simulink model "ballInaHoop_trajStab"  (R2017a)
settings: Solver=ode45  StartTime=0.0  StopTime=15  MaxStep=1e-3  RelTol=1e-3  EnableMultiTasking=on
undefined symbols (not defined in the file): Dpsi0, Dth0, prms, psi0, th0
libraries: simulink x1
settings Model: Creator=gurtnmar  LastModifiedBy=marti
settings SolverCC: AlgebraicLoopSolver=LineSearch
settings DataIOCC: LimitDataPoints=on  SaveFormat=Array
settings OptimizationCC: LifeSpan=inf
settings DebuggingCC: SFUnexpectedBacktrackingDiag=warning  SFNoUnconditionalDefaultTransitionDiag=warning  SFExecutionAtInitializationDiag=none
settings HardwareCC: ProdBitPerPointer=32  ProdBitPerSizeT=32  ProdBitPerPtrDiffT=32  ProdLargestAtomicFloat=None  ProdIntDivRoundTo=Undefined  ProdEndianess=Unspecified  ProdWordSize=32  ProdHWDeviceType=32-bit Generic
settings ModelReferenceCC: PropagateSignalLabelsOutOfModel=off
settings GRTTargetCC: TargetLangStandard=C89/C90 (ANSI)  GeneratePreprocessorConditionals=Disable all
settings ConfigComp: CovMetricSettings=dw  CovHtmlReporting=on  CovSaveCumulativeToWorkspaceVar=on  CovSaveSingleToWorkspaceVar=on  CovExternalEMLEnable=off

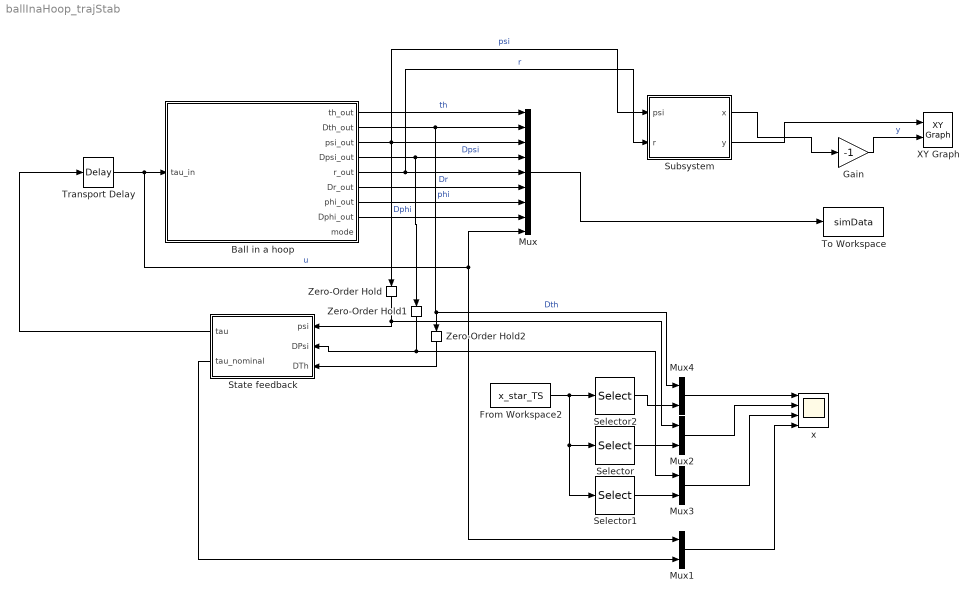
== system ballInaHoop_trajStab ==
  Ball in a hoop : Stateflow chart  TreatAsAtomicUnit=on
  From Workspace2 : FromWorkspace  VariableName=x_star_TS  SampleTime=prms.Ts  Interpolate=off  OutputAfterFinalValue=Setting to zero
  Gain : Gain  Gain=-1
  Mux : Mux  Inputs=9
  Mux{1..4} (4 alike) : Mux  Inputs=2
  Selector : Selector  InputPortWidth=3  IndexOptions=Index vector (dialog)  Indices=2  OutputSizes=1
  Selector1 : Selector  InputPortWidth=3  IndexOptions=Index vector (dialog)  Indices=3  OutputSizes=1
  Selector2 : Selector  InputPortWidth=3  IndexOptions=Index vector (dialog)  Indices=1  OutputSizes=1
  State feedback : Subsystem
  Subsystem : Subsystem
  To Workspace : ToWorkspace  VariableName=simData  SaveFormat=Timeseries  SampleTime=-1
  Transport Delay : TransportDelay  DelayTime=1/1000
  XY Graph : simulink/Sinks/XY Graph  xmin=-1.1*prms.Ro  xmax=1.1*prms.Ro  ymin=-1.1*prms.Ro  ymax=1.1*prms.Ro  st=-1
  Zero-Order Hold : ZeroOrderHold  SampleTime=prms.Ts
  Zero-Order Hold1 : ZeroOrderHold  SampleTime=prms.Ts
  Zero-Order Hold2 : ZeroOrderHold  SampleTime=prms.Ts
  x : Scope  NumInputPorts=4
  wires:
  Gain/1 -> XY Graph/2  "y"
  Mux/1 -> To Workspace/1
  Subsystem/2(y) -> XY Graph/1
  Subsystem/1(x) -> Gain/1
  Transport Delay/1 -> Ball in a hoop/1(tau_in), Mux/9, Mux1/1  "u"
  Ball in a hoop/1(th_out) -> Mux/1  "th"
  Ball in a hoop/2(Dth_out) -> Mux4/1, Zero-Order Hold2/1, Mux/2  "Dth"
  Ball in a hoop/3(psi_out) -> Zero-Order Hold/1, Subsystem/1(psi), Mux/3  "psi"
  Ball in a hoop/4(Dpsi_out) -> Zero-Order Hold1/1, Mux/4  "Dpsi"
  Ball in a hoop/5(r_out) -> Subsystem/2(r), Mux/5  "r"
  Ball in a hoop/6(Dr_out) -> Mux/6  "Dr"
  Ball in a hoop/7(phi_out) -> Mux/7  "phi"
  Ball in a hoop/8(Dphi_out) -> Mux/8  "Dphi"
  Zero-Order Hold1/1 -> Mux3/1, State feedback/2(DPsi)
  From Workspace2/1 -> Selector2/1, Selector1/1, Selector/1
  Selector/1 -> Mux2/2
  Selector1/1 -> Mux3/2
  Zero-Order Hold/1 -> Mux2/1, State feedback/1(psi)
  Mux4/1 -> x/1
  Mux2/1 -> x/2
  Mux3/1 -> x/3
  Selector2/1 -> Mux4/2
  Zero-Order Hold2/1 -> State feedback/3(DTh)
  Mux1/1 -> x/4
  State feedback/1(tau) -> Transport Delay/1
  State feedback/2(tau_nominal) -> Mux1/2

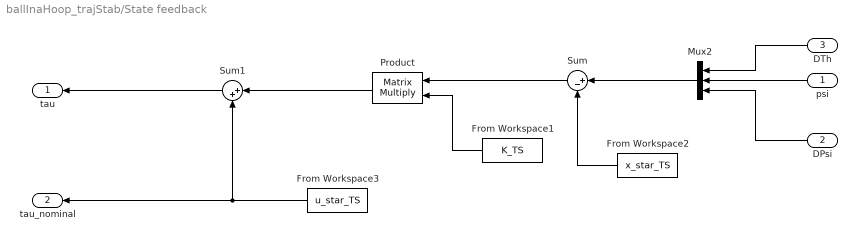
== system ballInaHoop_trajStab/State feedback ==
  psi : Inport
  DPsi : Inport  Port=2
  DTh : Inport  Port=3
  From Workspace1 : FromWorkspace  VariableName=K_TS  SampleTime=prms.Ts  Interpolate=off  OutputAfterFinalValue=Setting to zero
  From Workspace2 : FromWorkspace  VariableName=x_star_TS  SampleTime=prms.Ts  Interpolate=off  OutputAfterFinalValue=Setting to zero
  From Workspace3 : FromWorkspace  VariableName=u_star_TS  SampleTime=prms.Ts  Interpolate=off  OutputAfterFinalValue=Setting to zero
  Mux2 : Mux  Inputs=3
  Product : Product  Multiplication=Matrix(*)
  Sum : Sum  Inputs=|+-
  Sum1 : Sum  Inputs=|++
  tau : Outport
  tau_nominal : Outport  Port=2
  wires:
  From Workspace1/1 -> Product/2
  Mux2/1 -> Sum/1
  From Workspace2/1 -> Sum/2
  Sum1/1 -> tau/1
  psi/1 -> Mux2/2
  DPsi/1 -> Mux2/3
  Product/1 -> Sum1/1
  From Workspace3/1 -> Sum1/2, tau_nominal/1
  Sum/1 -> Product/1
  DTh/1 -> Mux2/1

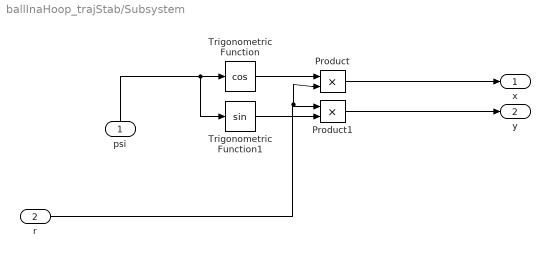
== system ballInaHoop_trajStab/Subsystem ==
  psi : Inport
  r : Inport  Port=2
  Product : Product
  Product1 : Product
  Trigonometric Function : Trigonometry  Operator=cos
  Trigonometric Function1 : Trigonometry
  x : Outport
  y : Outport  Port=2
  wires:
  Trigonometric Function/1 -> Product/1
  Product/1 -> x/1
  Product1/1 -> y/1
  Trigonometric Function1/1 -> Product1/2
  r/1 -> Product/2, Product1/1
  psi/1 -> Trigonometric Function1/1, Trigonometric Function/1

== stateflow chart ballInaHoop_trajStab/Ball in a hoop ==
  settings: updateMethod=CONTINUOUS
  state Free_fall
    du:
    th_dot = Dth;
    Dth_dot = prms.ath1*Dth + prms.bth*tau_in;
    phi_dot = Dphi;
    Dphi_dot = 0;
    r_dot = Dr;
    Dr_dot = r*Dpsi^2 + prms.g*cos(psi);
    psi_dot = Dpsi;
    Dpsi_dot = -(prms.g*sin(psi) + 2*Dpsi*Dr)/r;
    th_out = th;
    Dth_out = Dth;
    psi_out = psi;
    Dpsi_out = Dpsi;
    r_out = r;
    Dr_out = Dr;
    phi_out=phi;
    Dphi_out=Dphi;
    mode=2;
  state Ball_in_a_hoop
    du:
    th_dot = Dth;
    Dth_dot = prms.ath1*Dth + prms.ath2*sin(psi) + prms.ath3*Dpsi + prms.bth*tau_in;
    psi_dot = Dpsi;
    Dpsi_dot = prms.apsi1*Dth + prms.apsi2*sin(psi) + prms.apsi3*Dpsi + prms.bpsi*tau_in;
    th_out = th;
    Dth_out = Dth;
    psi_out = psi;
    Dpsi_out=Dpsi;
    phi_out=(th-psi)*prms.Ro/prms.Rb;
    Dphi_out = (Dth-Dpsi)*prms.Ro/prms.Rb;
    r_out = r;
    Dr_out = 0;
    mode=1;
  state Ball_on_the_inner_hoop
    du:
    th_dot = Dth;
    Dth_dot = prms.ath1*Dth + prms.bth*tau_in;
    psi_dot = Dpsi;
    Dpsi_dot = 1 / prms.in.a_bar * (-prms.in.b_bar*Dpsi ...
    - prms.in.c_bar*sin(psi) - prms.in.d_bar*Dth + prms.in.e_bar*tau_in);
    th_out = th;
    Dth_out = Dth;
    psi_out = psi;
    Dpsi_out=Dpsi;
    r_out = r;
    Dr_out = 0;
    phi_out= -(th-psi)*(prms.Ri/prms.Rb);
    Dphi_out = -(Dth-Dpsi)*(prms.Ri/prms.Rb);
    mode=3;
  (default) -> Ball_in_a_hoop : {
      | th=th0;
      | Dth=Dth0;
      | psi=psi0;
      | Dpsi=Dpsi0;
      | r = prms.Ro-prms.Rb;
      | }
  Ball_in_a_hoop -> Free_fall : [(-prms.g*cos(psi)-(prms.Ro-prms.Rb)*Dpsi^2)>eps]
      | {
      | phi = (th-psi)*prms.Ro/prms.Rb;
      | Dphi = (prms.Ro+prms.Rb)/prms.Rb*Dth - prms.Ro/prms.Rb*Dpsi;
      | r = (prms.Ro-prms.Rb);
      | Dr = 0;
      | }
  Ball_on_the_inner_hoop -> Free_fall : [(prms.g*cos(psi)+(prms.Ri+prms.Rb)*Dpsi^2) > eps]
      | {
      | phi = -(th-psi)*prms.Ri/prms.Rb;
      | Dphi = -((prms.Ri-prms.Rb)/prms.Rb*Dth - prms.Ri/prms.Rb*Dpsi);
      | r = (prms.Ri+prms.Rb);
      | Dr = 0;
      | }
  Free_fall -> Ball_on_the_inner_hoop [order 2] : [prms.Ri + prms.Rb - r > eps]
      | {
      | Dpsi = Dth+prms.Rb/prms.Ri*Dphi +Dpsi;
      | Dr = 0;
      | r = prms.Ri+prms.Rb
      | }
  Free_fall -> Ball_in_a_hoop [order 1] : [r - prms.Ro + prms.Rb > eps]
      | {
      | Dpsi = Dth - prms.Rb/prms.Ro*Dphi +Dpsi;
      | Dr = 0;
      | r = prms.Ro-prms.Rb
      | }
  data: th local; Dth local size=1; psi local size=1; Dpsi local size=1; phi local size=1; Dphi local size=1; th_out output size=1; Dth_out output; psi_out output; Dpsi_out output; r_out output; Dr_out output; tau_in input size=1; prms parameter; phi_out output; Dphi_out output; psi0 parameter; Dth0 parameter; th0 parameter; Dpsi0 parameter; mode output; Dr local; r local
  data th settings: updateMethod=SF_CONTINUOUS_TIME_DATA
  data Dth settings: updateMethod=SF_CONTINUOUS_TIME_DATA
  data psi settings: updateMethod=SF_CONTINUOUS_TIME_DATA
  data Dpsi settings: updateMethod=SF_CONTINUOUS_TIME_DATA
  data phi settings: updateMethod=SF_CONTINUOUS_TIME_DATA
  data Dphi settings: updateMethod=SF_CONTINUOUS_TIME_DATA
  data Dr settings: updateMethod=SF_CONTINUOUS_TIME_DATA
  data r settings: updateMethod=SF_CONTINUOUS_TIME_DATA
